simulink model "state_flow"  (R2019b)
settings: Solver=VariableStepAuto  StartTime=0.0  StopTime=10.0  RelTol=1e-3
settings Model: Creator=yangy  LastModifiedBy=yangy

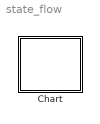
== system state_flow ==
  Chart : Stateflow chart  BlockKeywords=__PRM__SERIALIZED__DATA__:Stateflow Chart,Stateflow Diagram  TreatAsAtomicUnit=on

== stateflow chart state_flow/Chart ==
  state A
  state B
  (default) -> A
  B -> A : [e1]
  A -> B : {e1}
